simulink library "RGPBasedRealTimeControl_ayaz"  (R2018b)
settings: Solver=VariableStepAuto  StartTime=0.0  StopTime=10.0  RelTol=1e-3
undefined symbols (not defined in the file): postVarCtrlGain
libraries: filteredPDController_ul x3, RGPbasedSetpointControl x1, constantSetpoints_cl x1, slrtlib x1, squareWave_ul x1
settings Model: Creator=Ayaz  LastModifiedBy=Ayaz
settings DataIOCC: ReturnWorkspaceOutputs=on

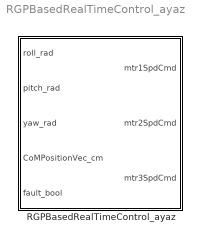
== system RGPBasedRealTimeControl_ayaz ==
  RGPBasedRealTimeControl_ayaz : Subsystem

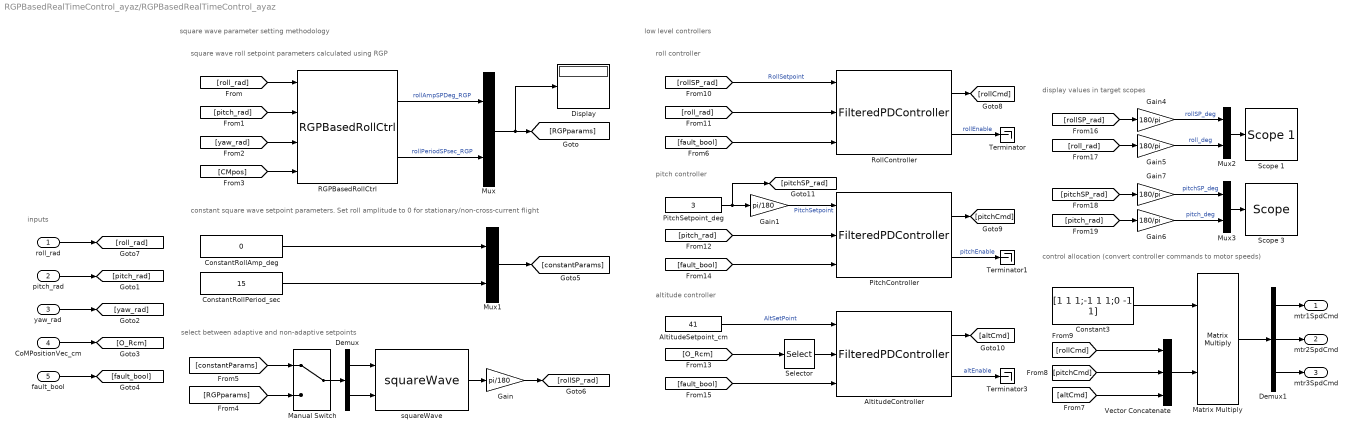
== system RGPBasedRealTimeControl_ayaz/RGPBasedRealTimeControl_ayaz ==
  note: display values in target scopes
  note: control allocation (convert controller commands to motor speeds)
  note: low level controllers
  note: altitude controller
  note: pitch controller
  note: roll controller
  note: select between adaptive and non-adaptive setpoints
  note: square wave parameter setting methodology
  note: constant square wave setpoint parameters. Set roll amplitude to 0 for stationary/non-cross-current flight
  note: square wave roll setpoint parameters calculated using RGP
  note: inputs
  roll_rad : Inport
  pitch_rad : Inport  Port=2
  yaw_rad : Inport  Port=3
  CoMPositionVec_cm : Inport  Port=4
  fault_bool : Inport  Port=5
  AltitudeController : filteredPDController_ul/FilteredPDController  enable=on  kp=0.1  kd=0  timeConstant_s=0.4  intialError=0  initialOutput=0
  AltitudeSetpoint_cm : Constant  Value=41
  Constant3 : Constant  Value=[1 1 1;-1 1 1;0 -1 1]
  ConstantRollAmp_deg : Constant  Value=0
  ConstantRollPeriod_sec : Constant  Value=15
  Demux : Demux  Outputs=2
  Demux1 : Demux  Outputs=3
  Display : Display
  Gain : Gain  Gain=pi/180
  Gain1 : Gain  Gain=pi/180
  Gain{4..7} (4 alike) : Gain  Gain=180/pi
  Manual Switch : ManualSwitch
  Matrix Multiply : Product  Multiplication=Matrix(*)
  Mux{,1..3} (4 alike) : Mux  Inputs=2
  PitchController : filteredPDController_ul/FilteredPDController  enable=on  kp=2.5  kd=1  timeConstant_s=0.15  intialError=0  initialOutput=0
  PitchSetpoint_deg : Constant  Value=3
  RGPBasedRollCtrl : RGPbasedSetpointControl/RGPBasedRollCtrl  FilterWindowSize=20  vRated=20  xBasis=basisVector  meanFcnProp=meanFcnProperties  meanFcnVec=meanFcnVector  hyperParams=hyperParameters  basisCovMat=basisCovMat  noiseVar=noiseVariance  predMeanGain=predMeanCtrlGain  postVarGain=2^postVarCtrlGain  initRollAmpDeg=0  initRollPeriodSec=20  ctrlTriggerInt=3
  RollController : filteredPDController_ul/FilteredPDController  enable=on  kp=5  kd=1  timeConstant_s=0.2  intialError=0  initialOutput=0
  Scope 1 : constantSetpoints_cl/ConstantSetpoints/Scope 1  scopeno=4  scopetype=Target  autostart=on  viewmode=Graphical rolling  formatstr='%15.6f'  grid=on  ylimits=30*[-1,1]  nosamples=1000  noprepostsamples=0  interleave=1  triggermode=FreeRun  triggersignal=1  trigsignalfromport=off  triggerlevel=0.0  triggerslope=Either  triggerscope=1  triggersample=0  filename=data.dat  mode=Lazy  writesize=512  autorestart=off  dynamicfilemode=off  maxwritefilesize=512*1024^2
  Scope 3 : slrtlib/Displays and Logging/Scope   scopeno=3  scopetype=Target  autostart=on  viewmode=Graphical rolling  formatstr='%15.6f'  grid=on  ylimits=20*[-1,1]  nosamples=1000  noprepostsamples=0  interleave=1  triggermode=FreeRun  triggersignal=1  trigsignalfromport=off  triggerlevel=0.0  triggerslope=Either  triggerscope=1  triggersample=0  filename=data.dat  mode=Lazy  writesize=512  autorestart=off  dynamicfilemode=off  maxwritefilesize=512*1024^2
  Selector : Selector  InputPortWidth=3  IndexOptions=Index vector (dialog)  Indices=3  OutputSizes=1
  Terminator : Terminator
  Terminator1 : Terminator
  Terminator3 : Terminator
  Vector Concatenate : Concatenate  NumInputs=3
  squareWave : squareWave_ul/squareWave  startDelay=4
  mtr1SpdCmd : Outport  VectorParamsAs1DForOutWhenUnconnected=off
  mtr2SpdCmd : Outport  Port=2  VectorParamsAs1DForOutWhenUnconnected=off
  mtr3SpdCmd : Outport  Port=3  VectorParamsAs1DForOutWhenUnconnected=off
  wires:
  Demux/1 -> squareWave/1
  Demux/2 -> squareWave/2
  Manual Switch/1 -> Demux/1
  roll_rad/1 -> [roll_rad]
  pitch_rad/1 -> [pitch_rad]
  yaw_rad/1 -> [yaw_rad]
  CoMPositionVec_cm/1 -> [O_Rcm]
  fault_bool/1 -> [fault_bool]
  [roll_rad] -> RGPBasedRollCtrl/1
  [pitch_rad] -> RGPBasedRollCtrl/2
  [yaw_rad] -> RGPBasedRollCtrl/3
  [CMpos] -> RGPBasedRollCtrl/4
  RGPBasedRollCtrl/1 -> Mux/1  "rollAmpSPDeg_RGP"
  RGPBasedRollCtrl/2 -> Mux/2  "rollPeriodSPsec_RGP"
  Mux/1 -> Display/1, [RGPparams]
  [RGPparams] -> Manual Switch/2
  ConstantRollAmp_deg/1 -> Mux1/1
  ConstantRollPeriod_sec/1 -> Mux1/2
  Mux1/1 -> [constantParams]
  [constantParams] -> Manual Switch/1
  squareWave/1 -> Gain/1
  Gain/1 -> [rollSP_rad]
  Demux1/1 -> mtr1SpdCmd/1
  [fault_bool] -> AltitudeController/3
  [O_Rcm] -> Selector/1
  AltitudeController/2 -> Terminator3/1  "altEnable"
  [roll_rad] -> RollController/2
  PitchController/2 -> Terminator1/1  "pitchEnable"
  Vector Concatenate/1 -> Matrix Multiply/2
  Selector/1 -> AltitudeController/2
  AltitudeSetpoint_cm/1 -> AltitudeController/1  "AltSetPoint"
  [altCmd] -> Vector Concatenate/3
  [fault_bool] -> PitchController/3
  [rollCmd] -> Vector Concatenate/1
  Constant3/1 -> Matrix Multiply/1
  [pitch_rad] -> PitchController/2
  Demux1/3 -> mtr3SpdCmd/1
  [pitchCmd] -> Vector Concatenate/2
  RollController/2 -> Terminator/1  "rollEnable"
  [fault_bool] -> RollController/3
  RollController/1 -> [rollCmd]
  Demux1/2 -> mtr2SpdCmd/1
  AltitudeController/1 -> [altCmd]
  PitchController/1 -> [pitchCmd]
  [rollSP_rad] -> RollController/1  "RollSetpoint"
  Gain1/1 -> PitchController/1  "PitchSetpoint"
  Matrix Multiply/1 -> Demux1/1
  PitchSetpoint_deg/1 -> [pitchSP_rad], Gain1/1
  Gain5/1 -> Mux2/2  "roll_deg"
  [roll_rad] -> Gain5/1
  Mux3/1 -> Scope 3/1
  Gain4/1 -> Mux2/1  "rollSP_deg"
  [rollSP_rad] -> Gain4/1
  Mux2/1 -> Scope 1/1
  [pitch_rad] -> Gain6/1
  [pitchSP_rad] -> Gain7/1
  Gain6/1 -> Mux3/2  "pitch_deg"
  Gain7/1 -> Mux3/1  "pitchSP_deg"
